simulink model "wirkungsplan_mdl"  (R2013b)
settings: Solver=ode45  StartTime=0.0  StopTime=1000  RelTol=1e-3
values from neighbouring files (symbols this model uses):
  a13_stepinit = 0    [wirkungsplan.m]
  a13_steptime = 0    [wirkungsplan.m]
  a13_stepvalue = 0    [wirkungsplan.m]
  a1_stepinit = 0    [wirkungsplan.m]
  a1_steptime = 0    [wirkungsplan.m]
  a1_stepvalue = 0    [wirkungsplan.m]
  a22_stepinit = 0    [wirkungsplan.m]
  a22_steptime = 0    [wirkungsplan.m]
  a22_stepvalue = 0    [wirkungsplan.m]
  a2_stepinit = 0    [wirkungsplan.m]
  a2_steptime = 0    [wirkungsplan.m]
  a2_stepvalue = 0    [wirkungsplan.m]
  a32_stepinit = 0    [wirkungsplan.m]
  a32_steptime = 0    [wirkungsplan.m]
  a32_stepvalue = 0    [wirkungsplan.m]
  a3_stepinit = 0    [wirkungsplan.m]
  a3_steptime = 0    [wirkungsplan.m]
  a3_stepvalue = 0    [wirkungsplan.m]
  AL = 5e-1    (= 0.5)    [wirkungsplan.m]
  AT = 154    [wirkungsplan.m]
  AV = 5e-1    (= 0.5)    [wirkungsplan.m]
  g = 981    [wirkungsplan.m]
  h1_initvalue = 0    [wirkungsplan.m]
  h2_initvalue = 0    [wirkungsplan.m]
  h3_initvalue = 0    [wirkungsplan.m]
  Q1_stepinit = 0    [wirkungsplan.m]
  Q1_steptime = 0    [wirkungsplan.m]
  Q1_stepvalue = 0    [wirkungsplan.m]
  Q2_stepinit = 0    [wirkungsplan.m]
  Q2_steptime = 0    [wirkungsplan.m]
  Q2_stepvalue = 0    [wirkungsplan.m]
settings Model: Creator=daniw  LastModifiedBy=daniw

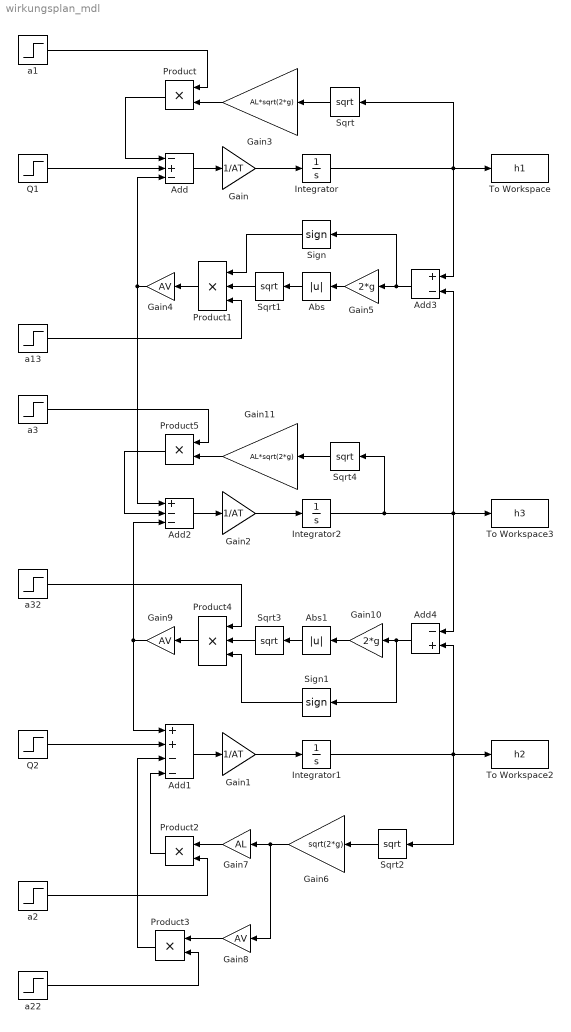
== system wirkungsplan_mdl ==
  Abs : Abs
  Abs1 : Abs
  Add : Sum  Inputs=-+-
  Add1 : Sum  Inputs=++--
  Add2 : Sum  Inputs=+--
  Add3 : Sum  Inputs=+-
  Add4 : Sum  Inputs=-+
  Gain : Gain  Gain=1/AT
  Gain1 : Gain  Gain=1/AT
  Gain10 : Gain  Gain=2*g
  Gain11 : Gain  Gain=AL*sqrt(2*g)
  Gain2 : Gain  Gain=1/AT
  Gain3 : Gain  Gain=AL*sqrt(2*g)
  Gain4 : Gain  Gain=AV
  Gain5 : Gain  Gain=2*g
  Gain6 : Gain  Gain=sqrt(2*g)
  Gain7 : Gain  Gain=AL
  Gain8 : Gain  Gain=AV
  Gain9 : Gain  Gain=AV
  Integrator : Integrator  InitialCondition=h1_initvalue
  Integrator1 : Integrator  InitialCondition=h2_initvalue
  Integrator2 : Integrator  InitialCondition=h3_initvalue
  Product{,2..3,5} (4 alike) : Product
  Product1 : Product  Inputs=3
  Product4 : Product  Inputs=3
  Q1 : Step  Time=Q1_steptime  Before=Q1_stepinit  After=Q1_stepvalue  SampleTime=0
  Q2 : Step  Time=Q2_steptime  Before=Q2_stepinit  After=Q2_stepvalue  SampleTime=0
  Sign : Signum
  Sign1 : Signum
  Sqrt{,1..4} (5 alike) : Sqrt  SaturateOnIntegerOverflow=on
  To Workspace : ToWorkspace  VariableName=h1  SampleTime=-1  SaveFormat=Structure With Time
  To Workspace2 : ToWorkspace  VariableName=h2  SampleTime=-1  SaveFormat=Structure With Time
  To Workspace3 : ToWorkspace  VariableName=h3  SampleTime=-1  SaveFormat=Structure With Time
  a1 : Step  Time=a1_steptime  Before=a1_stepinit  After=a1_stepvalue  SampleTime=0
  a13 : Step  Time=a13_steptime  Before=a13_stepinit  After=a13_stepvalue  SampleTime=0
  a2 : Step  Time=a2_steptime  Before=a2_stepinit  After=a2_stepvalue  SampleTime=0
  a22 : Step  Time=a22_steptime  Before=a22_stepinit  After=a22_stepvalue  SampleTime=0
  a3 : Step  Time=a3_steptime  Before=a3_stepinit  After=a3_stepvalue  SampleTime=0
  a32 : Step  Time=a32_steptime  Before=a32_stepinit  After=a32_stepvalue  SampleTime=0
  wires:
  Q1/1 -> Add/2
  Add/1 -> Gain/1
  Gain/1 -> Integrator/1
  Q2/1 -> Add1/2
  Add1/1 -> Gain1/1
  Gain1/1 -> Integrator1/1
  Add2/1 -> Gain2/1
  Gain2/1 -> Integrator2/1
  Product/1 -> Add/1
  Gain3/1 -> Product/2
  Sqrt/1 -> Gain3/1
  Integrator/1 -> To Workspace/1, Add3/1, Sqrt/1
  a1/1 -> Product/1
  Product1/1 -> Gain4/1
  Gain4/1 -> Add2/1, Add/3
  a13/1 -> Product1/3
  Sign/1 -> Product1/1
  Integrator2/1 -> Sqrt4/1, To Workspace3/1, Add3/2, Add4/1
  Add3/1 -> Gain5/1, Sign/1
  Gain5/1 -> Abs/1
  Abs/1 -> Sqrt1/1
  Sqrt1/1 -> Product1/2
  Integrator1/1 -> Add4/2, To Workspace2/1, Sqrt2/1
  Sqrt2/1 -> Gain6/1
  a2/1 -> Product2/2
  Gain6/1 -> Gain8/1, Gain7/1
  Gain7/1 -> Product2/1
  Gain8/1 -> Product3/1
  a22/1 -> Product3/2
  Product2/1 -> Add1/4
  Product3/1 -> Add1/3
  Product4/1 -> Gain9/1
  Sign1/1 -> Product4/3
  Add4/1 -> Sign1/1, Gain10/1
  Gain10/1 -> Abs1/1
  Abs1/1 -> Sqrt3/1
  Sqrt3/1 -> Product4/2
  Gain9/1 -> Add1/1, Add2/3
  a32/1 -> Product4/1
  Gain11/1 -> Product5/2
  Sqrt4/1 -> Gain11/1
  a3/1 -> Product5/1
  Product5/1 -> Add2/2
